simulink model "shem2_2"  (R2023a)
settings: Solver=VariableStepAuto  StartTime=0.0  StopTime=10.0  RelTol=1e-3
settings Model: Creator=fynjy  LastModifiedBy=fynjy

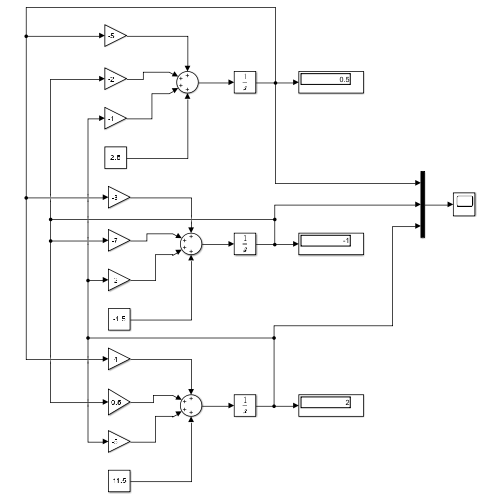
[thumbnail: Simulink's stored preview of the top-level diagram]
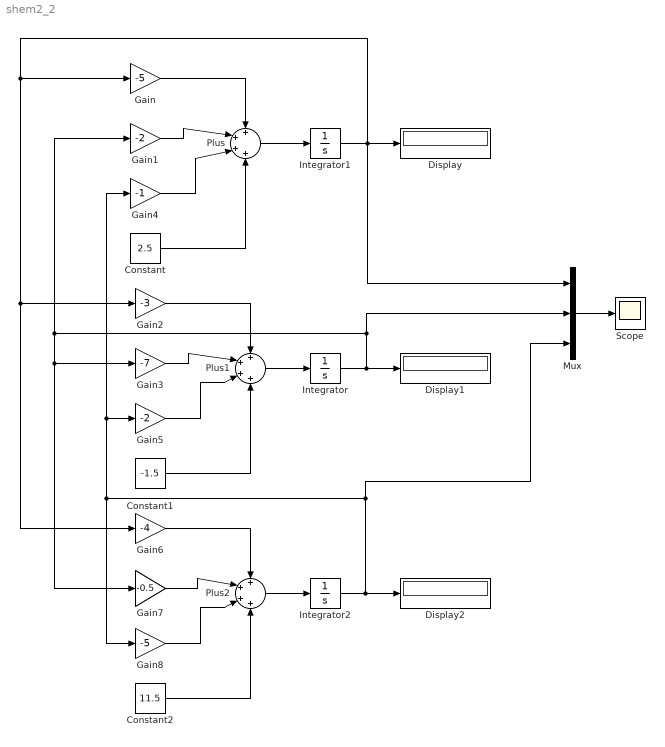
== system shem2_2 ==
  Constant : Constant  Value=2.5
  Constant1 : Constant  Value=-1.5
  Constant2 : Constant  Value=11.5
  Display : Display
  Display1 : Display
  Display2 : Display
  Gain : Gain  Gain=-5
  Gain1 : Gain  Gain=-2
  Gain2 : Gain  Gain=-3
  Gain3 : Gain  Gain=-7
  Gain4 : Gain  Gain=-1
  Gain5 : Gain  Gain=-2
  Gain6 : Gain  Gain=-4
  Gain7 : Gain  Gain=-0.5
  Gain8 : Gain  Gain=-5
  Integrator : Integrator
  Integrator1 : Integrator
  Integrator2 : Integrator
  Mux : Mux  Inputs=3
  Plus : Sum  Inputs=++++
  Plus1 : Sum  Inputs=++++
  Plus2 : Sum  Inputs=++++
  Scope : Scope
  wires:
  Integrator1/1 -> Gain/1, Gain2/1, Gain6/1, Mux/1, Display/1
  Plus/1 -> Integrator1/1
  Gain1/1 -> Plus/2
  Gain/1 -> Plus/1
  Integrator/1 -> Mux/2, Gain7/1, Gain3/1, Gain1/1, Display1/1
  Mux/1 -> Scope/1
  Constant/1 -> Plus/4
  Gain4/1 -> Plus/3
  Plus1/1 -> Integrator/1
  Constant1/1 -> Plus1/4
  Gain3/1 -> Plus1/2
  Gain2/1 -> Plus1/1
  Gain5/1 -> Plus1/3
  Plus2/1 -> Integrator2/1
  Gain6/1 -> Plus2/1
  Gain8/1 -> Plus2/3
  Gain7/1 -> Plus2/2
  Constant2/1 -> Plus2/4
  Integrator2/1 -> Mux/3, Gain4/1, Gain5/1, Gain8/1, Display2/1
